simulink model "structure"  (R2012b)
settings: Solver=FixedStepDiscrete  StartTime=0.0  StopTime=10.0  FixedStep=delta_t  RelTol=1e-3
undefined symbols (not defined in the file): ca1, ca2, ca3, ca4, cb, D, delta_t, Ixx, Iyy, Izz, m, S_pinv, sa1, sa2, sa3, sa4, sb
settings Model: Creator=Kerianne  LastModifiedBy=Kerianne
settings DataIOCC: SaveFormat=Structure
settings OptimizationCC: InlineParams=on

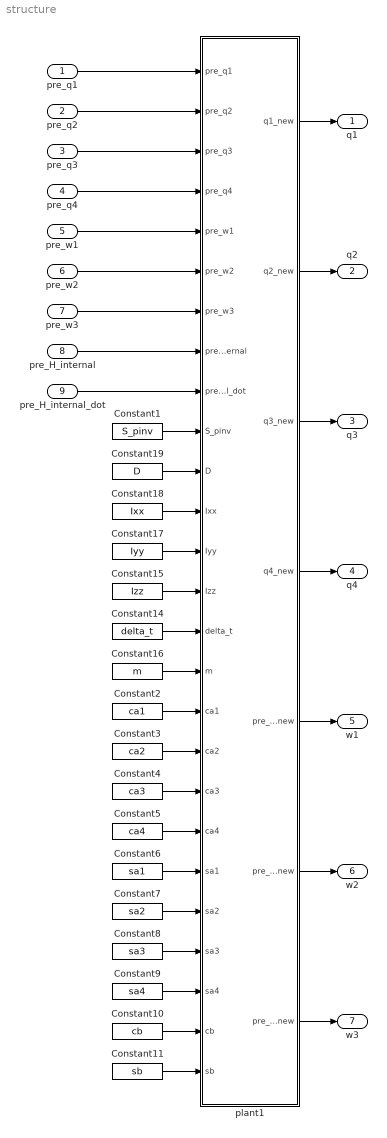
== system structure ==
  pre_q1 : Inport
  pre_q2 : Inport  Port=2
  pre_q3 : Inport  Port=3
  pre_q4 : Inport  Port=4
  pre_w1 : Inport  Port=5
  pre_w2 : Inport  Port=6
  pre_w3 : Inport  Port=7
  pre_H_internal : Inport  Port=8  PortDimensions=3
  pre_H_internal_dot : Inport  Port=9  PortDimensions=3
  Constant1 : Constant  Value=S_pinv
  Constant10 : Constant  Value=cb
  Constant11 : Constant  Value=sb
  Constant14 : Constant  Value=delta_t
  Constant15 : Constant  Value=Izz
  Constant16 : Constant  Value=m
  Constant17 : Constant  Value=Iyy
  Constant18 : Constant  Value=Ixx
  Constant19 : Constant  Value=D
  Constant2 : Constant  Value=ca1
  Constant3 : Constant  Value=ca2
  Constant4 : Constant  Value=ca3
  Constant5 : Constant  Value=ca4
  Constant6 : Constant  Value=sa1
  Constant7 : Constant  Value=sa2
  Constant8 : Constant  Value=sa3
  Constant9 : Constant  Value=sa4
  plant1 : MATLAB Function  TreatAsAtomicUnit=on
  q1 : Outport
  q2 : Outport  Port=2
  q3 : Outport  Port=3
  q4 : Outport  Port=4
  w1 : Outport  Port=5
  w2 : Outport  Port=6
  w3 : Outport  Port=7
  wires:
  plant1/1(q1_new) -> q1/1
  plant1/2(q2_new) -> q2/1
  plant1/3(q3_new) -> q3/1
  plant1/4(q4_new) -> q4/1
  plant1/5(pre_w1_new) -> w1/1
  plant1/6(pre_w2_new) -> w2/1
  plant1/7(pre_w3_new) -> w3/1
  Constant14/1 -> plant1/15(delta_t)
  Constant19/1 -> plant1/11(D)
  Constant18/1 -> plant1/12(Ixx)
  Constant17/1 -> plant1/13(Iyy)
  Constant15/1 -> plant1/14(Izz)
  pre_w3/1 -> plant1/7(pre_w3)
  pre_w2/1 -> plant1/6(pre_w2)
  pre_w1/1 -> plant1/5(pre_w1)
  pre_q4/1 -> plant1/4(pre_q4)
  pre_q3/1 -> plant1/3(pre_q3)
  pre_q2/1 -> plant1/2(pre_q2)
  pre_q1/1 -> plant1/1(pre_q1)
  Constant16/1 -> plant1/16(m)
  pre_H_internal_dot/1 -> plant1/9(pre_H_internal_dot)
  pre_H_internal/1 -> plant1/8(pre_H_internal)
  Constant1/1 -> plant1/10(S_pinv)
  Constant6/1 -> plant1/21(sa1)
  Constant5/1 -> plant1/20(ca4)
  Constant4/1 -> plant1/19(ca3)
  Constant3/1 -> plant1/18(ca2)
  Constant2/1 -> plant1/17(ca1)
  Constant11/1 -> plant1/26(sb)
  Constant10/1 -> plant1/25(cb)
  Constant9/1 -> plant1/24(sa4)
  Constant8/1 -> plant1/23(sa3)
  Constant7/1 -> plant1/22(sa2)

== matlab function structure/plant1 ==
  data: pre_q1 input; pre_q2 input; pre_q3 input; pre_q4 input; pre_w1 input; pre_w2 input; pre_w3 input; pre_H_internal input; pre_H_internal_dot input; S_pinv input; q1_new output; D input; Ixx input; Iyy input; Izz input; delta_t input; q2_new output; q3_new output; q4_new output; pre_w1_new output; pre_w2_new output; pre_w3_new output; m input; ca1 input; ca2 input; ca3 input; ca4 input; sa1 input; sa2 input; sa3 input; sa4 input; cb input; sb input
function  [q1_new,q2_new,q3_new,q4_new,pre_w1_new,pre_w2_new,pre_w3_new]= fcn(pre_q1,pre_q2,pre_q3,pre_q4,pre_w1,pre_w2,pre_w3,pre_H_internal,pre_H_internal_dot,S_pinv,D,Ixx,Iyy,Izz,delta_t,m,ca1,ca2,ca3,ca4,sa1,sa2,sa3,sa4,cb,sb)

% ca1,ca2,ca3,ca4,sa1,sa2,sa3,sa4,cb,sb

pre_psi = S_pinv*pre_H_internal;  
psi_1 = pre_psi(1);
psi_2 = pre_psi(2);
psi_3 = pre_psi(3);
psi_4 = pre_psi(4);
psi_dot = S_pinv*pre_H_internal_dot;
psi_dot_1 = psi_dot(1);
psi_dot_2 = psi_dot(2);
psi_dot_3 = psi_dot(3);
psi_dot_4 = psi_dot(4);
m1 = m(1);
m3 = m(2);
m2 = m(3);

%RWA angle rates
q1_dot = (pre_q2*pre_w3)/2 - (pre_q3*pre_w2)/2 + (pre_q4*pre_w1)/2;
q2_dot = (pre_q3*pre_w1)/2 - (pre_q1*pre_w3)/2 + (pre_q4*pre_w2)/2;
q3_dot = (pre_q1*pre_w2)/2 - (pre_q2*pre_w1)/2 + (pre_q4*pre_w3)/2;
q4_dot = - (pre_q1*pre_w1)/2 - (pre_q2*pre_w2)/2 - (pre_q3*pre_w3)/2;
pre_w1_dot = m1/Ixx - psi_2*((D*pre_w2*cb)/Ixx - (D*pre_w3*sa2*sb)/Ixx) - psi_3*((D*pre_w2*cb)/Ixx - (D*pre_w3*sa3*sb)/Ixx) - psi_4*((D*pre_w2*cb)/Ixx - (D*pre_w3*sa4*sb)/Ixx) - psi_1*((D*pre_w2*cb)/Ixx - (D*pre_w3*sa1*sb)/Ixx) + (Iyy*pre_w2*pre_w3)/Ixx - (Izz*pre_w2*pre_w3)/Ixx + (D*psi_dot_1*ca1*sb)/Ixx + (D*psi_dot_2*ca2*sb)/Ixx + (D*psi_dot_3*ca3*sb)/Ixx + (D*psi_dot_4*ca4*sb)/Ixx;
pre_w2_dot = psi_1*((D*pre_w1*cb)/Iyy + (D*pre_w3*ca1*sb)/Iyy) + psi_2*((D*pre_w1*cb)/Iyy + (D*pre_w3*ca2*sb)/Iyy) + psi_3*((D*pre_w1*cb)/Iyy + (D*pre_w3*ca3*sb)/Iyy) + psi_4*((D*pre_w1*cb)/Iyy + (D*pre_w3*ca4*sb)/Iyy) + m2/Iyy - (Ixx*pre_w1*pre_w3)/Iyy + (Izz*pre_w1*pre_w3)/Iyy - (D*psi_dot_1*sa1*sb)/Iyy - (D*psi_dot_2*sa2*sb)/Iyy - (D*psi_dot_3*sa3*sb)/Iyy - (D*psi_dot_4*sa4*sb)/Iyy;
pre_w3_dot = m3/Izz - psi_1*((D*pre_w2*ca1*sb)/Izz + (D*pre_w1*sa1*sb)/Izz) - psi_2*((D*pre_w2*ca2*sb)/Izz + (D*pre_w1*sa2*sb)/Izz) - psi_3*((D*pre_w2*ca3*sb)/Izz + (D*pre_w1*sa3*sb)/Izz) - psi_4*((D*pre_w2*ca4*sb)/Izz + (D*pre_w1*sa4*sb)/Izz) + (Ixx*pre_w1*pre_w2)/Izz - (Iyy*pre_w1*pre_w2)/Izz - (D*psi_dot_1*cb)/Izz - (D*psi_dot_2*cb)/Izz - (D*psi_dot_3*cb)/Izz - (D*psi_dot_4*cb)/Izz;
   
% Update individual states
q1_new = pre_q1+q1_dot*delta_t;
q2_new = pre_q2+q2_dot*delta_t;
q3_new = pre_q3+q3_dot*delta_t;
q4_new = pre_q4+q4_dot*delta_t;
pre_w1_new = pre_w1+pre_w1_dot*delta_t;
pre_w2_new = pre_w2+pre_w2_dot*delta_t;
pre_w3_new = pre_w3+pre_w3_dot*delta_t;
